simulink model "gm_sampleModel2005_1_sub"  (R2023a)
settings: Solver=VariableStepAuto  StartTime=0.0  StopTime=10.0  RelTol=1e-3
libraries: simulink x1
settings Model: Creator=user1  LastModifiedBy=user1
settings OptimizationCC: BlockReduction=off  ConditionallyExecuteInputs=off
settings DebuggingCC: InheritedTsInSrcMsg=none

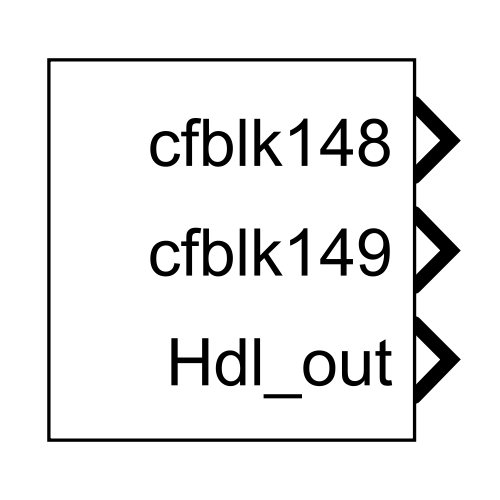
[thumbnail: Simulink's stored preview of the top-level diagram]
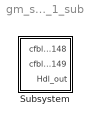
== system gm_sampleModel2005_1_sub ==
  Subsystem : Subsystem

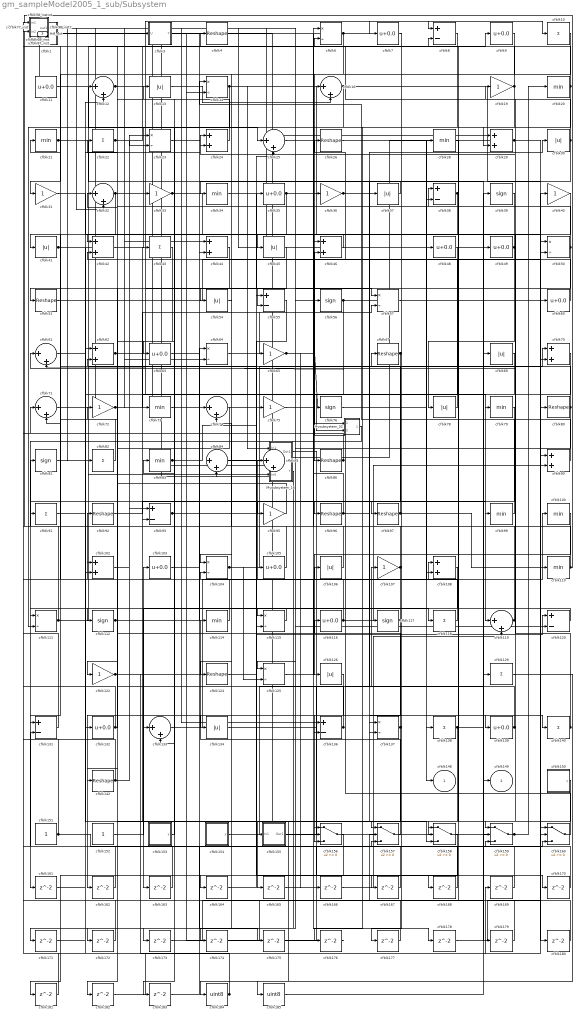
== system gm_sampleModel2005_1_sub/Subsystem ==
  Mysubsystem_16 : Subsystem
  Mysubsystem_32 : Subsystem
  cfblk1 : Subsystem  mask(Detect Fall Negative){vinit=double(0), InputProcessing=Elements as channels (sample based), OutDataTypeStr=uint8}
      mask prompts: vinit "Simulink:masks:InitialCondition_MP"; InputProcessing "Simulink:masks:InputProcessing_MP"; OutDataTypeStr "Simulink:masks:OutputDataType_MP"
      mask help: Simulink:masks:DetectFallNegative_MD
      mask init:
      | InputProcessing = 'Elements as channels (sample based)';
      | OutDataTypeStr = 'uint8';
      | vinit = double(0);
      mask TypeOptions InputProcessing: Simulink:masks:ColumnsAsChannelsFrameBased | Simulink:masks:ElementsAsChannelsSampleBased
      mask TypeOptions OutDataTypeStr: Simulink:masks:uint8 | Simulink:masks:boolean
      mask Display: fprintf('U < 0\n&  NOT\nU/z < 0')
  cfblk{10,22,43,82,91,118,129,138,140} (9 alike) : Sum  Inputs=+  OutDataTypeStr=uint8
  cfblk{20..21,28,34,73,79,83,99..100,110,114} (11 alike) : MinMax  OutDataTypeStr=uint8
  cfblk101_inst : Subsystem
  cfblk{24,29,42,44,46,62,70,90,102,108} (10 alike) : Sum  OutDataTypeStr=uint8
  cfblk{7,9,11,35,48..49,60,63,103,105,116,132,139} (13 alike) : Bias  Bias=0.0  SaturateOnIntegerOverflow=off
  cfblk{6,14,23,50,57,64,104,111,115,125,137} (11 alike) : Product  Inputs=*/  OutDataTypeStr=uint8  RndMeth=Zero  SaturateOnIntegerOverflow=on
  cfblk{13,30,37,41,45,54,69,78,106,126,134} (11 alike) : Abs  OutDataTypeStr=uint8  SaturateOnIntegerOverflow=off
  cfblk{19,31,33,36,40,65,72,75,95,107,122} (11 alike) : Gain  OutDataTypeStr=uint8
  cfblk109_inst : Subsystem
  cfblk{39,56,76,81,112,117} (6 alike) : Signum
  cfblk{12,16,25,32,61,71,74,84..85,119,133} (11 alike) : Sum  Inputs=|++  OutDataTypeStr=uint8
  cfblk{8,38,55,93,120,131,136} (7 alike) : Sum  Inputs=+-  OutDataTypeStr=uint8
  cfblk121_inst : Subsystem
  cfblk123_inst : Subsystem
  cfblk{4,26,51,67,80,86,92,96..97,124,142} (11 alike) : Reshape
  cfblk128_inst : Subsystem
  cfblk135_inst : Subsystem
  cfblk150 : Subsystem  mask(Counter Free-Running){NumBits=double(16), tsamp=double(-1)}
      mask prompts: NumBits "Simulink:masks:NumberOfBits_MP"; tsamp "Simulink:masks:SampleTime_MP"
      mask help: Simulink:masks:CounterFreeRunning_MD
  cfblk151 : Constant  OutDataTypeStr=uint8  SampleTime=-1
  cfblk152 : Constant  OutDataTypeStr=uint8  SampleTime=-1
  cfblk153 : Subsystem  mask(Counter Free-Running){NumBits=double(16), tsamp=double(-1)}
      mask prompts: NumBits "Simulink:masks:NumberOfBits_MP"; tsamp "Simulink:masks:SampleTime_MP"
      mask help: Simulink:masks:CounterFreeRunning_MD
  cfblk154 : Subsystem  mask(Counter Free-Running){NumBits=double(16), tsamp=double(-1)}
      mask prompts: NumBits "Simulink:masks:NumberOfBits_MP"; tsamp "Simulink:masks:SampleTime_MP"
      mask help: Simulink:masks:CounterFreeRunning_MD
  cfblk155 : Subsystem
  cfblk{156..160} (5 alike) : Switch  OutDataTypeStr=uint8  SaturateOnIntegerOverflow=off  InputSameDT=off
  cfblk15_inst : Subsystem
  cfblk{161..183} (23 alike) : Delay  SampleTime=1
  cfblk184 : DataTypeConversion  OutDataTypeStr=uint8  SaturateOnIntegerOverflow=off  RndMeth=Floor
  cfblk185 : DataTypeConversion  OutDataTypeStr=uint8  SaturateOnIntegerOverflow=off  RndMeth=Floor
  cfblk18_inst : Subsystem
  cfblk27_inst : Subsystem
  cfblk3 : Subsystem  mask(Detect Fall Nonpositive){vinit=double(0), InputProcessing=Elements as channels (sample based), OutDataTypeStr=uint8}
      mask prompts: vinit "Simulink:masks:InitialCondition_MP"; InputProcessing "Simulink:masks:InputProcessing_MP"; OutDataTypeStr "Simulink:masks:OutputDataType_MP"
      mask help: Simulink:masks:DetectFallNonpositive_MD
      mask init:
      | InputProcessing = 'Elements as channels (sample based)';
      | OutDataTypeStr = 'uint8';
      | vinit = double(0);
      mask TypeOptions InputProcessing: Simulink:masks:ColumnsAsChannelsFrameBased | Simulink:masks:ElementsAsChannelsSampleBased
      mask TypeOptions OutDataTypeStr: Simulink:masks:uint8 | Simulink:masks:boolean
      mask Display: fprintf('U <= 0\n&  NOT\nU/z <= 0')
  cfblk53_inst : Subsystem
  cfblk58_inst : Subsystem
  cfblk68_inst : Subsystem
  cfblk77_inst : Subsystem
  cfblk87_inst : Subsystem
  cfblk98_inst : Subsystem
  cfblk148 : Outport  OutDataTypeStr=uint8  SampleTime=1  VectorParamsAs1DForOutWhenUnconnected=off
  cfblk149 : Outport  Port=2  OutDataTypeStr=uint8  SampleTime=1  VectorParamsAs1DForOutWhenUnconnected=off
  Hdl_out : Outport  Port=3  OutDataTypeStr=uint8  SampleTime=1
  wires:
  Mysubsystem_16/1(Out1) -> cfblk170/1
  Mysubsystem_16/2(Y) -> cfblk173/1
  Mysubsystem_32/1(Out1) -> cfblk161/1
  cfblk1/1(Y) -> cfblk8/1, cfblk55/2, cfblk6/2
  cfblk10/1 -> cfblk86/1
  cfblk100/1 -> cfblk126/1
  cfblk101_inst/1(out1) -> cfblk64/2, cfblk73/1
  cfblk102/1 -> cfblk93/1
  cfblk103/1 -> cfblk64/1
  cfblk104/1 -> cfblk70/1, cfblk125/2
  cfblk105/1 -> cfblk83/1
  cfblk106/1 -> cfblk81/1
  cfblk107/1 -> cfblk6/1, cfblk104/2
  cfblk108/1 -> cfblk163/1
  cfblk109_inst/1(out1) -> cfblk85/2
  cfblk11/1 -> cfblk25/1
  cfblk110/1 -> cfblk53_inst/1(in1), cfblk128_inst/2(in2)
  cfblk111/1 -> cfblk4/1, cfblk18_inst/1(in1), Mysubsystem_16/4(In5)
  cfblk112/1 -> cfblk84/2, cfblk100/1
  cfblk114/1 -> cfblk98_inst/2(in2)
  cfblk115/1 -> cfblk111/1
  cfblk116/1 -> cfblk90/2, cfblk71/2, cfblk18_inst/2(in2)
  cfblk117/1 -> cfblk92/1, cfblk156/3
  cfblk118/1 -> cfblk21/1
  cfblk119/1 -> cfblk74/2, cfblk123_inst/1(in1), cfblk109_inst/2(in2)
  cfblk12/1 -> cfblk119/1, Mysubsystem_32/2(In2)
  cfblk120/1 -> cfblk112/1
  cfblk121_inst/1(out1) -> cfblk48/1, cfblk27_inst/2(in2), cfblk75/1
  cfblk122/1 -> cfblk169/1, cfblk28/1
  cfblk123_inst/1(out1) -> cfblk44/1
  cfblk124/1 -> cfblk35/1
  cfblk125/1 -> cfblk108/1
  cfblk126/1 -> cfblk162/1
  cfblk128_inst/1(out1) -> cfblk74/1
  cfblk129/1 -> cfblk184/1
  cfblk13/1 -> cfblk16/2
  cfblk131/1 -> cfblk58_inst/1(in1)
  cfblk132/1 -> cfblk62/2, cfblk101_inst/1(in1)
  cfblk133/1 -> cfblk85/1
  cfblk134/1 -> cfblk107/1
  cfblk135_inst/1(out1) -> cfblk82/1
  cfblk136/1 -> cfblk42/2, cfblk32/1
  cfblk137/1 -> cfblk102/1, cfblk172/1
  cfblk138/1 -> cfblk69/1, cfblk165/1
  cfblk139/1 -> cfblk46/2, cfblk106/1
  cfblk14/1 -> Mysubsystem_32/1(In1), cfblk149/1, Mysubsystem_16/1(In1), cfblk43/1
  cfblk140/1 -> cfblk61/1, cfblk24/1
  cfblk142/1 -> cfblk121_inst/1(in1), cfblk23/1
  cfblk15_inst/1(out1) -> cfblk3/1(U)
  cfblk150/1(y) -> cfblk185/1
  cfblk151/1 -> cfblk27_inst/1(in1), cfblk160/3
  cfblk152/1 -> cfblk103/1
  cfblk153/1(y) -> cfblk13/1
  cfblk154/1(y) -> cfblk39/1
  cfblk155/1(Out1) -> cfblk37/1
  cfblk156/1 -> cfblk181/1
  cfblk157/1 -> cfblk114/1
  cfblk158/1 -> cfblk164/1
  cfblk159/1 -> Hdl_out/1, cfblk20/1
  cfblk16/1 -> cfblk44/2, cfblk160/2
  cfblk160/1 -> cfblk116/1
  cfblk161/1 -> cfblk12/2
  cfblk162/1 -> cfblk98_inst/1(in1)
  cfblk163/1 -> cfblk68_inst/1(in1)
  cfblk164/1 -> cfblk120/1
  cfblk165/1 -> cfblk70/2
  cfblk166/1 -> cfblk119/2
  cfblk167/1 -> cfblk123_inst/2(in2)
  cfblk168/1 -> cfblk131/2
  cfblk169/1 -> cfblk157/3
  cfblk170/1 -> cfblk38/1
  cfblk171/1 -> cfblk24/2
  cfblk172/1 -> cfblk58_inst/2(in2)
  cfblk173/1 -> cfblk157/2
  cfblk174/1 -> cfblk159/2
  cfblk175/1 -> cfblk90/1
  cfblk176/1 -> cfblk1/1(U)
  cfblk177/1 -> cfblk135_inst/2(in2)
  cfblk178/1 -> cfblk50/2
  cfblk179/1 -> cfblk8/2
  cfblk18_inst/1(out1) -> cfblk29/1
  cfblk180/1 -> cfblk77_inst/2(in2)
  cfblk181/1 -> cfblk101_inst/2(in2)
  cfblk182/1 -> cfblk160/1
  cfblk183/1 -> cfblk159/3
  cfblk184/1 -> cfblk87_inst/2(in2), cfblk62/1
  cfblk185/1 -> cfblk129/1
  cfblk19/1 -> cfblk68_inst/2(in2), cfblk133/2, cfblk109_inst/1(in1), cfblk111/2
  cfblk20/1 -> cfblk77_inst/1(in1), cfblk29/2
  cfblk21/1 -> cfblk179/1, cfblk148/1
  cfblk22/1 -> cfblk9/1, cfblk23/2
  cfblk23/1 -> cfblk175/1
  cfblk24/1 -> cfblk135_inst/1(in1)
  cfblk25/1 -> cfblk137/1
  cfblk26/1 -> cfblk140/1
  cfblk27_inst/1(out1) -> cfblk7/1
  cfblk28/1 -> cfblk158/2
  cfblk29/1 -> cfblk80/1, Mysubsystem_16/2(In2)
  cfblk3/1(Y) -> cfblk57/1
  cfblk30/1 -> cfblk15_inst/2(in2), cfblk137/2
  cfblk31/1 -> cfblk45/1
  cfblk32/1 -> cfblk131/1, cfblk33/1
  cfblk33/1 -> cfblk117/1, cfblk108/2
  cfblk34/1 -> cfblk56/1
  cfblk35/1 -> cfblk63/1, cfblk180/1
  cfblk36/1 -> cfblk30/1, cfblk158/3
  cfblk37/1 -> cfblk34/1
  cfblk38/1 -> cfblk125/1, cfblk104/1
  cfblk39/1 -> cfblk136/2
  cfblk4/1 -> cfblk38/2
  cfblk40/1 -> cfblk159/1
  cfblk41/1 -> Mysubsystem_16/3(In3), cfblk79/1
  cfblk42/1 -> cfblk156/1
  cfblk43/1 -> cfblk122/1
  cfblk44/1 -> cfblk51/1
  cfblk45/1 -> cfblk182/1
  cfblk46/1 -> cfblk41/1
  cfblk48/1 -> cfblk176/1
  cfblk49/1 -> cfblk78/1, cfblk42/1
  cfblk50/1 -> cfblk128_inst/1(in1), cfblk155/1(In1)
  cfblk51/1 -> cfblk40/1
  cfblk53_inst/1(out1) -> cfblk11/1
  cfblk54/1 -> cfblk124/1
  cfblk55/1 -> cfblk105/1
  cfblk56/1 -> cfblk61/2, cfblk174/1, cfblk115/1
  cfblk57/1 -> cfblk50/1
  cfblk58_inst/1(out1) -> cfblk60/1
  cfblk6/1 -> cfblk31/1, cfblk10/1
  cfblk60/1 -> cfblk22/1
  cfblk61/1 -> cfblk102/2
  cfblk62/1 -> cfblk115/2, cfblk99/1
  cfblk63/1 -> cfblk157/1
  cfblk64/1 -> cfblk16/1
  cfblk65/1 -> cfblk76/1, cfblk166/1
  cfblk67/1 -> cfblk134/1, cfblk91/1
  cfblk68_inst/1(out1) -> cfblk49/1, cfblk121_inst/2(in2)
  cfblk69/1 -> cfblk158/1
  cfblk7/1 -> cfblk177/1
  cfblk70/1 -> cfblk93/2
  cfblk71/1 -> cfblk55/1
  cfblk72/1 -> cfblk57/2, cfblk118/1
  cfblk73/1 -> cfblk133/1
  cfblk74/1 -> cfblk142/1
  cfblk75/1 -> cfblk178/1
  cfblk76/1 -> cfblk138/1
  cfblk77_inst/1(out1) -> cfblk136/1
  cfblk78/1 -> cfblk26/1
  cfblk79/1 -> cfblk95/1
  cfblk8/1 -> cfblk96/1
  cfblk80/1 -> cfblk53_inst/2(in2), cfblk171/1
  cfblk81/1 -> cfblk132/1
  cfblk82/1 -> cfblk87_inst/1(in1)
  cfblk83/1 -> cfblk25/2, cfblk183/1
  cfblk84/1 -> cfblk46/1
  cfblk85/1 -> cfblk84/1
  cfblk86/1 -> cfblk71/1, cfblk15_inst/1(in1)
  cfblk87_inst/1(out1) -> cfblk32/2, cfblk12/1
  cfblk9/1 -> cfblk54/1
  cfblk90/1 -> cfblk19/1
  cfblk91/1 -> cfblk156/2
  cfblk92/1 -> cfblk97/1
  cfblk93/1 -> cfblk65/1, cfblk168/1, cfblk167/1, cfblk14/2
  cfblk95/1 -> cfblk72/1
  cfblk96/1 -> cfblk139/1, cfblk36/1
  cfblk97/1 -> cfblk67/1, cfblk110/1
  cfblk98_inst/1(out1) -> cfblk120/2
  cfblk99/1 -> cfblk14/1

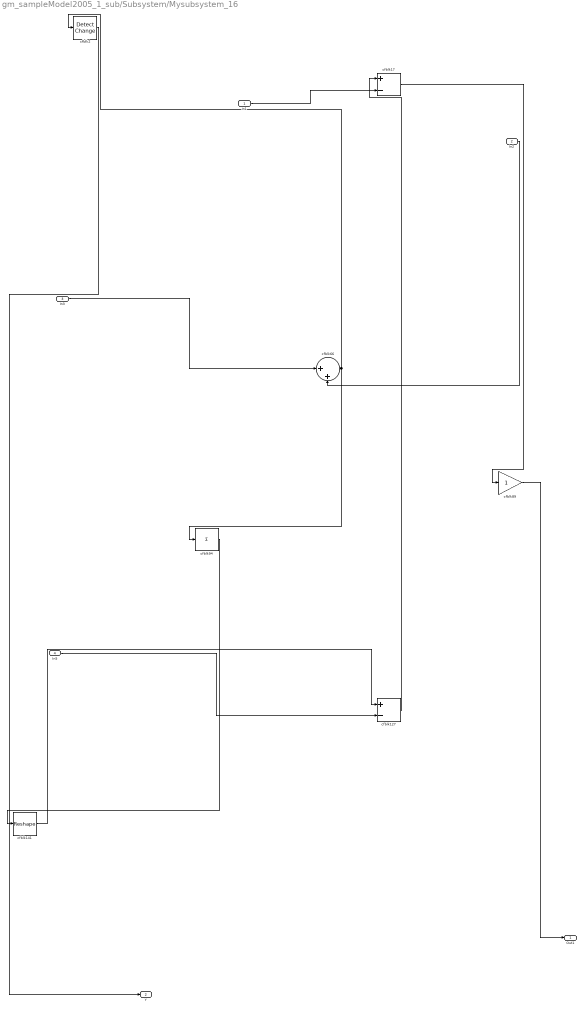
== system gm_sampleModel2005_1_sub/Subsystem/Mysubsystem_16 ==
  In1 : Inport  OutDataTypeStr=uint8  PortDimensions=1  SampleTime=1
  In2 : Inport  Port=2  OutDataTypeStr=uint8  PortDimensions=1  SampleTime=1
  In3 : Inport  Port=3  OutDataTypeStr=uint8  PortDimensions=1  SampleTime=1
  In5 : Inport  Port=4  OutDataTypeStr=uint8  PortDimensions=1  SampleTime=1
  cfblk127 : Sum  Inputs=+-
  cfblk141 : Reshape
  cfblk17 : Sum  Inputs=+-
  cfblk2 : simulink/Logic and Bit Operations/Detect Change  vinit=0  OutDataTypeStr=boolean
      settings: LibrarySourceBlock=|
      | hdlsllib/Logic and Bit
      | Operations/Detect
      | Change
  cfblk66 : Sum  Inputs=|++
  cfblk89 : Gain
  cfblk94 : Sum  Inputs=+
  Out1 : Outport  SampleTime=1
  Y : Outport  Port=2  SampleTime=1
  wires:
  In1/1 -> cfblk17/2
  In2/1 -> cfblk66/2
  In3/1 -> cfblk66/1
  In5/1 -> cfblk127/2
  cfblk127/1 -> cfblk17/1
  cfblk141/1 -> cfblk127/1
  cfblk17/1 -> cfblk89/1
  cfblk2/1 -> Y/1
  cfblk66/1 -> cfblk2/1, cfblk94/1
  cfblk89/1 -> Out1/1
  cfblk94/1 -> cfblk141/1

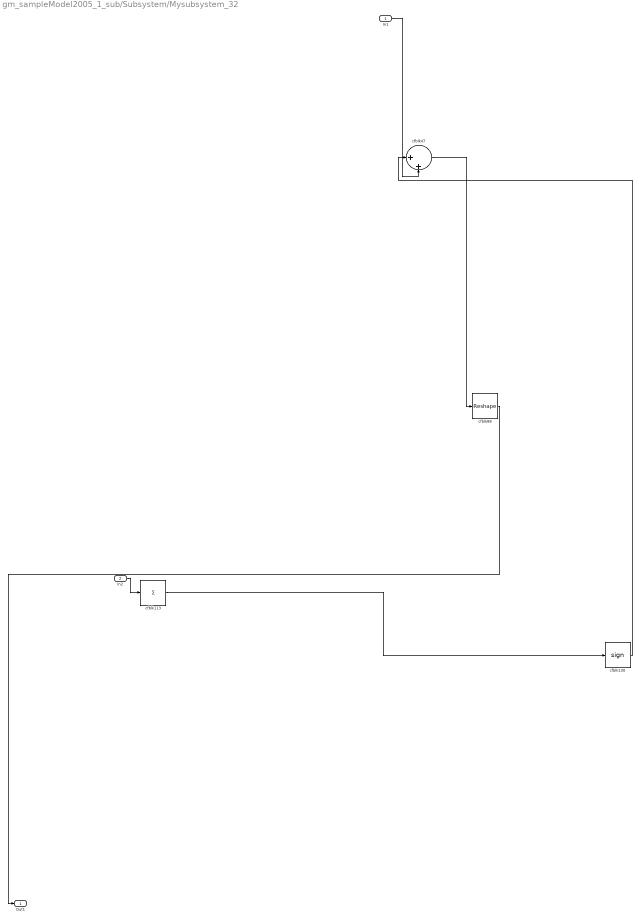
== system gm_sampleModel2005_1_sub/Subsystem/Mysubsystem_32 ==
  In1 : Inport  OutDataTypeStr=uint8  PortDimensions=1  SampleTime=1
  In2 : Inport  Port=2  OutDataTypeStr=uint8  PortDimensions=1  SampleTime=1
  cfblk113 : Sum  Inputs=+
  cfblk130 : Signum
  cfblk47 : Sum  Inputs=|++
  cfblk88 : Reshape
  Out1 : Outport  SampleTime=1
  wires:
  In1/1 -> cfblk47/2
  In2/1 -> cfblk113/1
  cfblk113/1 -> cfblk130/1
  cfblk130/1 -> cfblk47/1
  cfblk47/1 -> cfblk88/1
  cfblk88/1 -> Out1/1

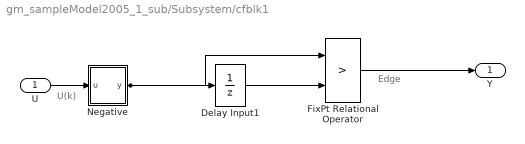
== system gm_sampleModel2005_1_sub/Subsystem/cfblk1 ==
  note: U(k)
  note: Edge
  U : Inport  OutDataTypeStr=uint8  SampleTime=1
  Delay Input1 : UnitDelay  Description=Store in Global RAM  DisableCoverage=on  InitialCondition=vinit  SampleTime=-1  HasFrameUpgradeWarning=on
  FixPt Relational Operator : RelationalOperator  Operator=>  OutDataTypeStr=fixdt(0, 8)  ZeroCross=off  InputSameDT=off
  Negative : Subsystem  mask(Compare To Zero){relop=<, OutDataTypeStr=boolean, ZeroCross=off}
      mask prompts: relop "Simulink:masks:Operator_MP"; OutDataTypeStr "Simulink:masks:OutputDataType_MP"; ZeroCross "Simulink:masks:EnableZerocrossingDetection_MP"
      mask help: Simulink:masks:CompareToZero_MD
      mask init:
      | OutDataTypeStr = 'boolean';
      | ZeroCross = 'off';
      | blkName = 'sampleModel2005_1_sub/Subsystem/cfblk1/Negative';
      | relop = '<';
      | setValue = 'boolean';
      mask TypeOptions relop: == | ~= | < | <= | >= | >
      mask TypeOptions OutDataTypeStr: Simulink:masks:uint8 | Simulink:masks:boolean
      mask Callback ZeroCross: sl('zeroCrossEnable', gcbh);
      mask Display: disp([relop,' 0'])
  Y : Outport  SampleTime=1
  wires:
  U/1 -> Negative/1(u)
  Delay Input1/1 -> FixPt Relational Operator/2
  FixPt Relational Operator/1 -> Y/1
  Negative/1(y) -> FixPt Relational Operator/1, Delay Input1/1

== system gm_sampleModel2005_1_sub/Subsystem/cfblk101_inst ==
  in1 : Inport  OutDataTypeStr=uint8  SampleTime=1
  in2 : Inport  Port=2  OutDataTypeStr=uint8  SampleTime=1
  mul_cfblk101_dotp_mulcomp : Product  Inputs=**  OutDataTypeStr=uint8  SampleTime=1
  out1 : Outport  OutDataTypeStr=uint8  SampleTime=1
  wires:
  in1/1 -> mul_cfblk101_dotp_mulcomp/1
  in2/1 -> mul_cfblk101_dotp_mulcomp/2
  mul_cfblk101_dotp_mulcomp/1 -> out1/1

== system gm_sampleModel2005_1_sub/Subsystem/cfblk109_inst ==
  in1 : Inport  OutDataTypeStr=uint8  SampleTime=1
  in2 : Inport  Port=2  OutDataTypeStr=uint8  SampleTime=1
  mul_cfblk109_dotp_mulcomp : Product  Inputs=**  OutDataTypeStr=uint8  SampleTime=1
  out1 : Outport  OutDataTypeStr=uint8  SampleTime=1
  wires:
  in1/1 -> mul_cfblk109_dotp_mulcomp/1
  in2/1 -> mul_cfblk109_dotp_mulcomp/2
  mul_cfblk109_dotp_mulcomp/1 -> out1/1

== system gm_sampleModel2005_1_sub/Subsystem/cfblk121_inst ==
  in1 : Inport  OutDataTypeStr=uint8  SampleTime=1
  in2 : Inport  Port=2  OutDataTypeStr=uint8  SampleTime=1
  mul_cfblk121_dotp_mulcomp : Product  Inputs=**  OutDataTypeStr=uint8  SampleTime=1
  out1 : Outport  OutDataTypeStr=uint8  SampleTime=1
  wires:
  in1/1 -> mul_cfblk121_dotp_mulcomp/1
  in2/1 -> mul_cfblk121_dotp_mulcomp/2
  mul_cfblk121_dotp_mulcomp/1 -> out1/1

== system gm_sampleModel2005_1_sub/Subsystem/cfblk123_inst ==
  in1 : Inport  OutDataTypeStr=uint8  SampleTime=1
  in2 : Inport  Port=2  OutDataTypeStr=uint8  SampleTime=1
  mul_cfblk123_dotp_mulcomp : Product  Inputs=**  OutDataTypeStr=uint8  SampleTime=1
  out1 : Outport  OutDataTypeStr=uint8  SampleTime=1
  wires:
  in1/1 -> mul_cfblk123_dotp_mulcomp/1
  in2/1 -> mul_cfblk123_dotp_mulcomp/2
  mul_cfblk123_dotp_mulcomp/1 -> out1/1

== system gm_sampleModel2005_1_sub/Subsystem/cfblk128_inst ==
  in1 : Inport  OutDataTypeStr=uint8  SampleTime=1
  in2 : Inport  Port=2  OutDataTypeStr=uint8  SampleTime=1
  mul_cfblk128_dotp_mulcomp : Product  Inputs=**  OutDataTypeStr=uint8  SampleTime=1
  out1 : Outport  OutDataTypeStr=uint8  SampleTime=1
  wires:
  in1/1 -> mul_cfblk128_dotp_mulcomp/1
  in2/1 -> mul_cfblk128_dotp_mulcomp/2
  mul_cfblk128_dotp_mulcomp/1 -> out1/1

== system gm_sampleModel2005_1_sub/Subsystem/cfblk135_inst ==
  in1 : Inport  OutDataTypeStr=uint8  SampleTime=1
  in2 : Inport  Port=2  OutDataTypeStr=uint8  SampleTime=1
  mul_cfblk135_dotp_mulcomp : Product  Inputs=**  OutDataTypeStr=uint8  SampleTime=1
  out1 : Outport  OutDataTypeStr=uint8  SampleTime=1
  wires:
  in1/1 -> mul_cfblk135_dotp_mulcomp/1
  in2/1 -> mul_cfblk135_dotp_mulcomp/2
  mul_cfblk135_dotp_mulcomp/1 -> out1/1

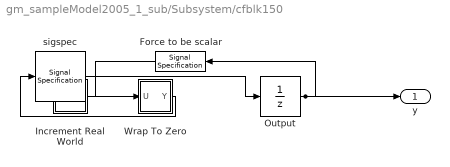
== system gm_sampleModel2005_1_sub/Subsystem/cfblk150 ==
  Force to be scalar : SignalSpecification  DisableCoverage=on  Dimensions=1
  Increment Real World : Subsystem  mask(Real World Value Increment){}
      mask help: Simulink:masks:RealWorldValueIncrement_MD
      mask Display: disp('V++')
  Output : UnitDelay  InitialCondition=0.0  SampleTime=tsamp  HasFrameUpgradeWarning=on
  Wrap To Zero : Subsystem  mask(Wrap To Zero){Threshold=double(65535)}
      mask prompts: Threshold "Simulink:masks:Threshold_MP"
      mask help: Simulink:masks:WrapToZero_MD
  sigspec : SignalSpecification  OutDataTypeStr=uint16  Dimensions=1
  y : Outport  SampleTime=1
  wires:
  Force to be scalar/1 -> Increment Real World/1(u)
  Increment Real World/1(y) -> Wrap To Zero/1(U)
  Output/1 -> Force to be scalar/1, y/1
  Wrap To Zero/1(Y) -> sigspec/1
  sigspec/1 -> Output/1

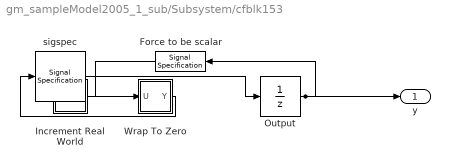
== system gm_sampleModel2005_1_sub/Subsystem/cfblk153 ==
  Force to be scalar : SignalSpecification  DisableCoverage=on  Dimensions=1
  Increment Real World : Subsystem  mask(Real World Value Increment){}
      mask help: Simulink:masks:RealWorldValueIncrement_MD
      mask Display: disp('V++')
  Output : UnitDelay  InitialCondition=0.0  SampleTime=tsamp  HasFrameUpgradeWarning=on
  Wrap To Zero : Subsystem  mask(Wrap To Zero){Threshold=double(65535)}
      mask prompts: Threshold "Simulink:masks:Threshold_MP"
      mask help: Simulink:masks:WrapToZero_MD
  sigspec : SignalSpecification  OutDataTypeStr=uint16  Dimensions=1
  y : Outport  SampleTime=1
  wires:
  Force to be scalar/1 -> Increment Real World/1(u)
  Increment Real World/1(y) -> Wrap To Zero/1(U)
  Output/1 -> Force to be scalar/1, y/1
  Wrap To Zero/1(Y) -> sigspec/1
  sigspec/1 -> Output/1

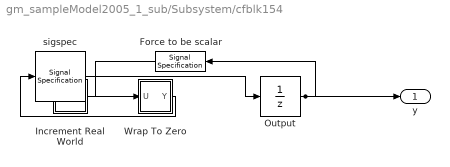
== system gm_sampleModel2005_1_sub/Subsystem/cfblk154 ==
  Force to be scalar : SignalSpecification  DisableCoverage=on  Dimensions=1
  Increment Real World : Subsystem  mask(Real World Value Increment){}
      mask help: Simulink:masks:RealWorldValueIncrement_MD
      mask Display: disp('V++')
  Output : UnitDelay  InitialCondition=0.0  SampleTime=tsamp  HasFrameUpgradeWarning=on
  Wrap To Zero : Subsystem  mask(Wrap To Zero){Threshold=double(65535)}
      mask prompts: Threshold "Simulink:masks:Threshold_MP"
      mask help: Simulink:masks:WrapToZero_MD
  sigspec : SignalSpecification  OutDataTypeStr=uint16  Dimensions=1
  y : Outport  SampleTime=1
  wires:
  Force to be scalar/1 -> Increment Real World/1(u)
  Increment Real World/1(y) -> Wrap To Zero/1(U)
  Output/1 -> Force to be scalar/1, y/1
  Wrap To Zero/1(Y) -> sigspec/1
  sigspec/1 -> Output/1

== system gm_sampleModel2005_1_sub/Subsystem/cfblk155 ==
  In1 : Inport  OutDataTypeStr=uint8  PortDimensions=1  SampleTime=1
  Out1 : Outport  SampleTime=1
  wires:
  In1/1 -> Out1/1

== system gm_sampleModel2005_1_sub/Subsystem/cfblk15_inst ==
  in1 : Inport  OutDataTypeStr=uint8  SampleTime=1
  in2 : Inport  Port=2  OutDataTypeStr=uint8  SampleTime=1
  mul_cfblk15_dotp_mulcomp : Product  Inputs=**  OutDataTypeStr=uint8  SampleTime=1
  out1 : Outport  OutDataTypeStr=uint8  SampleTime=1
  wires:
  in1/1 -> mul_cfblk15_dotp_mulcomp/1
  in2/1 -> mul_cfblk15_dotp_mulcomp/2
  mul_cfblk15_dotp_mulcomp/1 -> out1/1

== system gm_sampleModel2005_1_sub/Subsystem/cfblk18_inst ==
  in1 : Inport  OutDataTypeStr=uint8  SampleTime=1
  in2 : Inport  Port=2  OutDataTypeStr=uint8  SampleTime=1
  mul_cfblk18_dotp_mulcomp : Product  Inputs=**  OutDataTypeStr=uint8  SampleTime=1
  out1 : Outport  OutDataTypeStr=uint8  SampleTime=1
  wires:
  in1/1 -> mul_cfblk18_dotp_mulcomp/1
  in2/1 -> mul_cfblk18_dotp_mulcomp/2
  mul_cfblk18_dotp_mulcomp/1 -> out1/1

== system gm_sampleModel2005_1_sub/Subsystem/cfblk27_inst ==
  in1 : Inport  OutDataTypeStr=uint8  SampleTime=1
  in2 : Inport  Port=2  OutDataTypeStr=uint8  SampleTime=1
  mul_cfblk27_dotp_mulcomp : Product  Inputs=**  OutDataTypeStr=uint8  SampleTime=1
  out1 : Outport  OutDataTypeStr=uint8  SampleTime=1
  wires:
  in1/1 -> mul_cfblk27_dotp_mulcomp/1
  in2/1 -> mul_cfblk27_dotp_mulcomp/2
  mul_cfblk27_dotp_mulcomp/1 -> out1/1

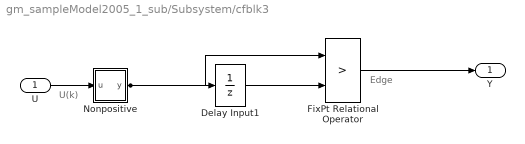
== system gm_sampleModel2005_1_sub/Subsystem/cfblk3 ==
  note: U(k)
  note: Edge
  U : Inport  OutDataTypeStr=uint8  SampleTime=1
  Delay Input1 : UnitDelay  Description=Store in Global RAM  DisableCoverage=on  InitialCondition=vinit  SampleTime=-1  HasFrameUpgradeWarning=on
  FixPt Relational Operator : RelationalOperator  Operator=>  OutDataTypeStr=fixdt(0, 8)  ZeroCross=off  InputSameDT=off
  Nonpositive : Subsystem  mask(Compare To Zero){relop=<=, OutDataTypeStr=boolean, ZeroCross=off}
      mask prompts: relop "Simulink:masks:Operator_MP"; OutDataTypeStr "Simulink:masks:OutputDataType_MP"; ZeroCross "Simulink:masks:EnableZerocrossingDetection_MP"
      mask help: Simulink:masks:CompareToZero_MD
      mask init:
      | OutDataTypeStr = 'boolean';
      | ZeroCross = 'off';
      | blkName = 'sampleModel2005_1_sub/Subsystem/cfblk3/Nonpositive';
      | relop = '<=';
      | setValue = 'boolean';
      mask TypeOptions relop: == | ~= | < | <= | >= | >
      mask TypeOptions OutDataTypeStr: Simulink:masks:uint8 | Simulink:masks:boolean
      mask Callback ZeroCross: sl('zeroCrossEnable', gcbh);
      mask Display: disp([relop,' 0'])
  Y : Outport  SampleTime=1
  wires:
  U/1 -> Nonpositive/1(u)
  Delay Input1/1 -> FixPt Relational Operator/2
  FixPt Relational Operator/1 -> Y/1
  Nonpositive/1(y) -> FixPt Relational Operator/1, Delay Input1/1

== system gm_sampleModel2005_1_sub/Subsystem/cfblk53_inst ==
  in1 : Inport  OutDataTypeStr=uint8  SampleTime=1
  in2 : Inport  Port=2  OutDataTypeStr=uint8  SampleTime=1
  mul_cfblk53_dotp_mulcomp : Product  Inputs=**  OutDataTypeStr=uint8  SampleTime=1
  out1 : Outport  OutDataTypeStr=uint8  SampleTime=1
  wires:
  in1/1 -> mul_cfblk53_dotp_mulcomp/1
  in2/1 -> mul_cfblk53_dotp_mulcomp/2
  mul_cfblk53_dotp_mulcomp/1 -> out1/1

== system gm_sampleModel2005_1_sub/Subsystem/cfblk58_inst ==
  in1 : Inport  OutDataTypeStr=uint8  SampleTime=1
  in2 : Inport  Port=2  OutDataTypeStr=uint8  SampleTime=1
  mul_cfblk58_dotp_mulcomp : Product  Inputs=**  OutDataTypeStr=uint8  SampleTime=1
  out1 : Outport  OutDataTypeStr=uint8  SampleTime=1
  wires:
  in1/1 -> mul_cfblk58_dotp_mulcomp/1
  in2/1 -> mul_cfblk58_dotp_mulcomp/2
  mul_cfblk58_dotp_mulcomp/1 -> out1/1

== system gm_sampleModel2005_1_sub/Subsystem/cfblk68_inst ==
  in1 : Inport  OutDataTypeStr=uint8  SampleTime=1
  in2 : Inport  Port=2  OutDataTypeStr=uint8  SampleTime=1
  mul_cfblk68_dotp_mulcomp : Product  Inputs=**  OutDataTypeStr=uint8  SampleTime=1
  out1 : Outport  OutDataTypeStr=uint8  SampleTime=1
  wires:
  in1/1 -> mul_cfblk68_dotp_mulcomp/1
  in2/1 -> mul_cfblk68_dotp_mulcomp/2
  mul_cfblk68_dotp_mulcomp/1 -> out1/1

== system gm_sampleModel2005_1_sub/Subsystem/cfblk77_inst ==
  in1 : Inport  OutDataTypeStr=uint8  SampleTime=1
  in2 : Inport  Port=2  OutDataTypeStr=uint8  SampleTime=1
  mul_cfblk77_dotp_mulcomp : Product  Inputs=**  OutDataTypeStr=uint8  SampleTime=1
  out1 : Outport  OutDataTypeStr=uint8  SampleTime=1
  wires:
  in1/1 -> mul_cfblk77_dotp_mulcomp/1
  in2/1 -> mul_cfblk77_dotp_mulcomp/2
  mul_cfblk77_dotp_mulcomp/1 -> out1/1

== system gm_sampleModel2005_1_sub/Subsystem/cfblk87_inst ==
  in1 : Inport  OutDataTypeStr=uint8  SampleTime=1
  in2 : Inport  Port=2  OutDataTypeStr=uint8  SampleTime=1
  mul_cfblk87_dotp_mulcomp : Product  Inputs=**  OutDataTypeStr=uint8  SampleTime=1
  out1 : Outport  OutDataTypeStr=uint8  SampleTime=1
  wires:
  in1/1 -> mul_cfblk87_dotp_mulcomp/1
  in2/1 -> mul_cfblk87_dotp_mulcomp/2
  mul_cfblk87_dotp_mulcomp/1 -> out1/1

== system gm_sampleModel2005_1_sub/Subsystem/cfblk98_inst ==
  in1 : Inport  OutDataTypeStr=uint8  SampleTime=1
  in2 : Inport  Port=2  OutDataTypeStr=uint8  SampleTime=1
  mul_cfblk98_dotp_mulcomp : Product  Inputs=**  OutDataTypeStr=uint8  SampleTime=1
  out1 : Outport  OutDataTypeStr=uint8  SampleTime=1
  wires:
  in1/1 -> mul_cfblk98_dotp_mulcomp/1
  in2/1 -> mul_cfblk98_dotp_mulcomp/2
  mul_cfblk98_dotp_mulcomp/1 -> out1/1

== system gm_sampleModel2005_1_sub/Subsystem/cfblk1/Negative ==
  u : Inport  OutDataTypeStr=uint8  SampleTime=1
  Compare : RelationalOperator  Operator=<  OutDataTypeStr=boolean  ZeroCross=off
  Constant : Constant  DisableCoverage=on  Value=0  OutDataTypeStr=Inherit: Inherit via back propagation  SampleTime=-1  PreserveConstantTs=on
  y : Outport  SampleTime=1
  wires:
  u/1 -> Compare/1
  Compare/1 -> y/1
  Constant/1 -> Compare/2

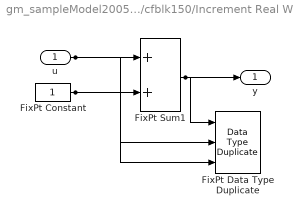
== system gm_sampleModel2005_1_sub/Subsystem/cfblk150/Increment Real World ==
  u : Inport  OutDataTypeStr=uint16  SampleTime=1
  FixPt Constant : Constant  DisableCoverage=on  OutDataTypeStr=Inherit: Inherit via back propagation  SampleTime=-1
  FixPt Data Type Duplicate : DataTypeDuplicate  DisableCoverage=on  NumInputPorts=3
  FixPt Sum1 : Sum  InputSameDT=on  OutDataTypeStr=Inherit: Inherit via back propagation  LockScale=on
  y : Outport  SampleTime=1
  wires:
  u/1 -> FixPt Sum1/1, FixPt Data Type Duplicate/2
  FixPt Constant/1 -> FixPt Sum1/2, FixPt Data Type Duplicate/3
  FixPt Sum1/1 -> FixPt Data Type Duplicate/1, y/1

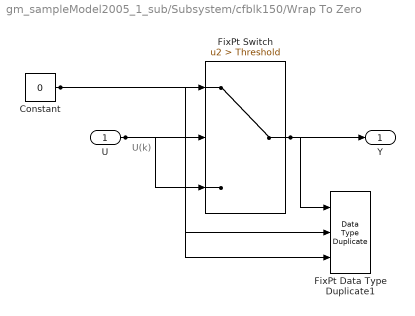
== system gm_sampleModel2005_1_sub/Subsystem/cfblk150/Wrap To Zero ==
  note: U(k)
  U : Inport  OutDataTypeStr=uint16  SampleTime=1
  Constant : Constant  DisableCoverage=on  Value=0  OutDataTypeStr=Inherit: Inherit via back propagation  SampleTime=-1
  FixPt Data Type Duplicate1 : DataTypeDuplicate  DisableCoverage=on  NumInputPorts=3
  FixPt Switch : Switch  Criteria=u2 > Threshold  Threshold=Threshold  OutDataTypeStr=Inherit: Inherit via back propagation  ZeroCross=off  SaturateOnIntegerOverflow=off  InputSameDT=off
  Y : Outport  SampleTime=1
  wires:
  U/1 -> FixPt Switch/3, FixPt Switch/2, FixPt Data Type Duplicate1/2
  Constant/1 -> FixPt Switch/1, FixPt Data Type Duplicate1/3
  FixPt Switch/1 -> FixPt Data Type Duplicate1/1, Y/1

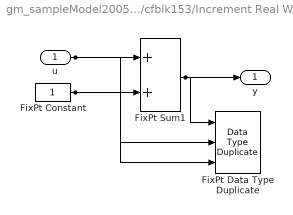
== system gm_sampleModel2005_1_sub/Subsystem/cfblk153/Increment Real World ==
  u : Inport  OutDataTypeStr=uint16  SampleTime=1
  FixPt Constant : Constant  DisableCoverage=on  OutDataTypeStr=Inherit: Inherit via back propagation  SampleTime=-1
  FixPt Data Type Duplicate : DataTypeDuplicate  DisableCoverage=on  NumInputPorts=3
  FixPt Sum1 : Sum  InputSameDT=on  OutDataTypeStr=Inherit: Inherit via back propagation  LockScale=on
  y : Outport  SampleTime=1
  wires:
  u/1 -> FixPt Sum1/1, FixPt Data Type Duplicate/2
  FixPt Constant/1 -> FixPt Sum1/2, FixPt Data Type Duplicate/3
  FixPt Sum1/1 -> FixPt Data Type Duplicate/1, y/1

== system gm_sampleModel2005_1_sub/Subsystem/cfblk153/Wrap To Zero ==
  note: U(k)
  U : Inport  OutDataTypeStr=uint16  SampleTime=1
  Constant : Constant  DisableCoverage=on  Value=0  OutDataTypeStr=Inherit: Inherit via back propagation  SampleTime=-1
  FixPt Data Type Duplicate1 : DataTypeDuplicate  DisableCoverage=on  NumInputPorts=3
  FixPt Switch : Switch  Criteria=u2 > Threshold  Threshold=Threshold  OutDataTypeStr=Inherit: Inherit via back propagation  ZeroCross=off  SaturateOnIntegerOverflow=off  InputSameDT=off
  Y : Outport  SampleTime=1
  wires:
  U/1 -> FixPt Switch/3, FixPt Switch/2, FixPt Data Type Duplicate1/2
  Constant/1 -> FixPt Switch/1, FixPt Data Type Duplicate1/3
  FixPt Switch/1 -> FixPt Data Type Duplicate1/1, Y/1

== system gm_sampleModel2005_1_sub/Subsystem/cfblk154/Increment Real World ==
  u : Inport  OutDataTypeStr=uint16  SampleTime=1
  FixPt Constant : Constant  DisableCoverage=on  OutDataTypeStr=Inherit: Inherit via back propagation  SampleTime=-1
  FixPt Data Type Duplicate : DataTypeDuplicate  DisableCoverage=on  NumInputPorts=3
  FixPt Sum1 : Sum  InputSameDT=on  OutDataTypeStr=Inherit: Inherit via back propagation  LockScale=on
  y : Outport  SampleTime=1
  wires:
  u/1 -> FixPt Sum1/1, FixPt Data Type Duplicate/2
  FixPt Constant/1 -> FixPt Sum1/2, FixPt Data Type Duplicate/3
  FixPt Sum1/1 -> FixPt Data Type Duplicate/1, y/1

== system gm_sampleModel2005_1_sub/Subsystem/cfblk154/Wrap To Zero ==
  note: U(k)
  U : Inport  OutDataTypeStr=uint16  SampleTime=1
  Constant : Constant  DisableCoverage=on  Value=0  OutDataTypeStr=Inherit: Inherit via back propagation  SampleTime=-1
  FixPt Data Type Duplicate1 : DataTypeDuplicate  DisableCoverage=on  NumInputPorts=3
  FixPt Switch : Switch  Criteria=u2 > Threshold  Threshold=Threshold  OutDataTypeStr=Inherit: Inherit via back propagation  ZeroCross=off  SaturateOnIntegerOverflow=off  InputSameDT=off
  Y : Outport  SampleTime=1
  wires:
  U/1 -> FixPt Switch/3, FixPt Switch/2, FixPt Data Type Duplicate1/2
  Constant/1 -> FixPt Switch/1, FixPt Data Type Duplicate1/3
  FixPt Switch/1 -> FixPt Data Type Duplicate1/1, Y/1

== system gm_sampleModel2005_1_sub/Subsystem/cfblk3/Nonpositive ==
  u : Inport  OutDataTypeStr=uint8  SampleTime=1
  Compare : RelationalOperator  Operator=<=  OutDataTypeStr=boolean  ZeroCross=off
  Constant : Constant  DisableCoverage=on  Value=0  OutDataTypeStr=Inherit: Inherit via back propagation  SampleTime=-1  PreserveConstantTs=on
  y : Outport  SampleTime=1
  wires:
  u/1 -> Compare/1
  Compare/1 -> y/1
  Constant/1 -> Compare/2
